simulink model "genMod"  (R2015b)
settings: Solver=VariableStepAuto  StartTime=0.0  StopTime=10.0  RelTol=1e-3
values from neighbouring files (symbols this model uses):
  D = diag(Y)    [init_power_system_v2_1.m]    (also in test1.m)
  sample_time_frr_a = 10    [init_power_system_v2_1.m]
undefined symbols (not defined in the file or in its folder): H, Ki, Kp, R, T_g, T_t
undefined symbols (not defined in the file): area_param_1
libraries: simulink x1
settings Model: Creator=tarje  LastModifiedBy=tarje

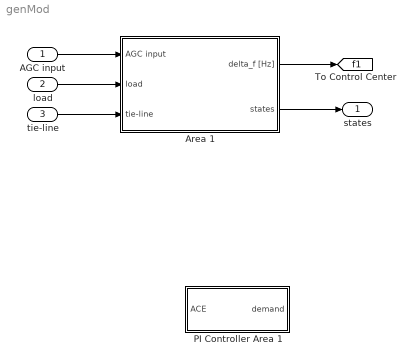
== system genMod ==
  AGC input : Inport
  load : Inport  Port=2
  tie-line : Inport  Port=3
  Area 1 : Subsystem  mask(Power system w/ primary control){param=area_param_1}
      mask prompts: param "Area parameters"
      mask help:
      | Linear model of generator, turbine and governor with primary control. All values are per unit delta values from a normal operating point.
      |
      | Parameters = [T_g T_t H D R]
      mask Display: % image('hydropower.jpg')
  PI Controller Area 1 : Subsystem  SystemSampleTime=sample_time_frr_a  mask(Secondary PI control){Kp=Kp(1), Ki=Ki(1)}
      mask help: Uses ace to estimate a demand for area. Gains should be negative.
  states : Outport
  tag scope: f1=global
  wires:
  AGC input/1 -> Area 1/1(AGC input)
  load/1 -> Area 1/2(load)
  tie-line/1 -> Area 1/3(tie-line)
  Area 1/2(states) -> states/1
  Area 1/1(delta_f [Hz]) -> [f1]

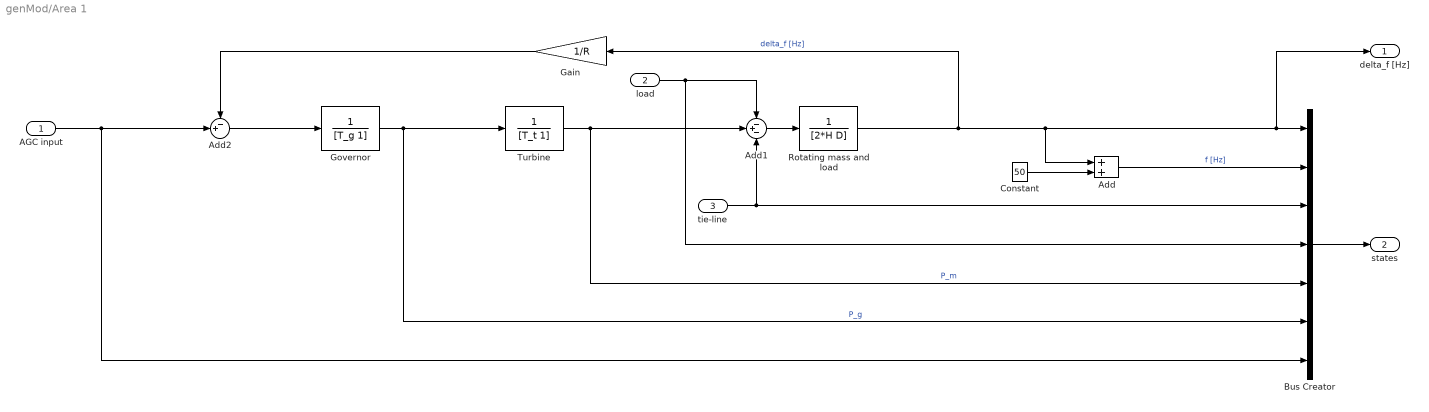
== system genMod/Area 1 ==
  AGC input : Inport
  load : Inport  Port=2
  tie-line : Inport  Port=3
  Add : Sum
  Add1 : Sum  Inputs=-+-
  Add2 : Sum  Inputs=-+|
  Bus Creator : BusCreator  Inputs=7
  Constant : Constant  Value=50
  Gain : Gain  Gain=1/R
  Governor : TransferFcn  Denominator=[T_g 1]
  Rotating mass and load : TransferFcn  Denominator=[2*H D]
  Turbine : TransferFcn  Denominator=[T_t 1]
  delta_f [Hz] : Outport
  states : Outport  Port=2
  wires:
  load/1 -> Bus Creator/4, Add1/1
  Bus Creator/1 -> states/1
  Turbine/1 -> Bus Creator/5, Add1/2  "P_m"
  Governor/1 -> Bus Creator/6, Turbine/1  "P_g"
  AGC input/1 -> Bus Creator/7, Add2/2
  tie-line/1 -> Add1/3, Bus Creator/3
  Constant/1 -> Add/2
  Add/1 -> Bus Creator/2  "f [Hz]"
  Add1/1 -> Rotating mass and load/1
  Gain/1 -> Add2/1
  Add2/1 -> Governor/1
  Rotating mass and load/1 -> Add/1, delta_f [Hz]/1, Bus Creator/1, Gain/1  "delta_f [Hz]"

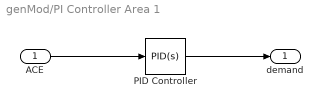
== system genMod/PI Controller Area 1 ==
  ACE : Inport
  PID Controller : simulink/Continuous/PID Controller  Controller=PID  TimeDomain=Continuous-time  SampleTime=-1  IntegratorMethod=Forward Euler  FilterMethod=Forward Euler  Form=Parallel  UseFilter=on  ControllerParametersSource=internal  P=Kp  I=Ki  D=0  N=0  InitialConditionSource=internal  InitialConditionForIntegrator=0  InitialConditionForFilter=0  ExternalReset=none  LimitOutput=off  UpperSaturationLimit=inf  LowerSaturationLimit=-inf  LinearizeAsGain=on  AntiWindupMode=none  Kb=1  TrackingMode=off  Kt=1  PParamMin=[]  PParamMax=[]  IParamMin=[]  IParamMax=[]  DParamMin=[]  DParamMax=[]  NParamMin=[]  NParamMax=[]  KbParamMin=[]  KbParamMax=[]  KtParamMin=[]  KtParamMax=[]  POutMin=[]  POutMax=[]  IOutMin=[]  IOutMax=[]  DOutMin=[]  DOutMax=[]  NOutMin=[]  NOutMax=[]  KbOutMin=[]  KbOutMax=[]  KtOutMin=[]  KtOutMax=[]  IntegratorOutMin=[]  IntegratorOutMax=[]  FilterOutMin=[]  FilterOutMax=[]  SumOutMin=[]  SumOutMax=[]  SumI1OutMin=[]  SumI1OutMax=[]  SumI2OutMin=[]  SumI2OutMax=[]  SumI3OutMin=[]  SumI3OutMax=[]  SumDOutMin=[]  SumDOutMax=[]  SaturationOutMin=[]  SaturationOutMax=[]  IntegratorContinuousStateAttributes=''  IntegratorStateMustResolveToSignalObject=off  IntegratorRTWStateStorageClass=Auto  FilterContinuousStateAttributes=''  FilterStateMustResolveToSignalObject=off  FilterRTWStateStorageClass=Auto  DifferentiatorICPrevScaledInput=0  DifferentiatorOutMin=[]  DifferentiatorOutMax=[]
  demand : Outport
  wires:
  PID Controller/1 -> demand/1
  ACE/1 -> PID Controller/1
